simulink model "CessnaCitationCitationIIModel550_Control"  (R2020b)
settings: Solver=FixedStepAuto  StartTime=0.0  StopTime=10.0  FixedStep=1e-12  MinStep=1e-12  RelTol=1
PreLoadFcn:
  | CessnaCitationData
  | datcom_data = datcomimport('Citation.out'); %Datcom data structures
InitFcn:
  | CessnaCitationData
values from neighbouring files (symbols this model uses):
  gnd_alt = -1500    [CessnaCitationData.m]
  inertia = [19990.488, -0.000, 7138.962 ... (first row only)    [CessnaCitationData.m]
  initpos_e = [0 0 -1500]    [CessnaCitationData.m]
  initrotrates_e = [0 0 0]    [CessnaCitationData.m]
  initrpy_e = [0 0 0]    [CessnaCitationData.m]
  initvel_b = [85 0 0]    [CessnaCitationData.m]
  mass = 3175    [CessnaCitationData.m]
  wind_angle_rates = [0 0 0]    [CessnaCitationData.m]
undefined symbols (not defined in the file or in its folder): Earth, m, s, WGS84
libraries: aerolibasang x4, aerolibtransform2 x4, simulink_extras x3, aerolibconvert2 x2, aerolibwind2 x1, aerolibatmos2 x1, shared3dof x1, sharedtransform x1, aerolibadyn x1
settings Model: SimulationMode=accelerator  Creator=pasquale  LastModifiedBy=pasquale
settings SolverCC: AutoInsertRateTranBlk=on

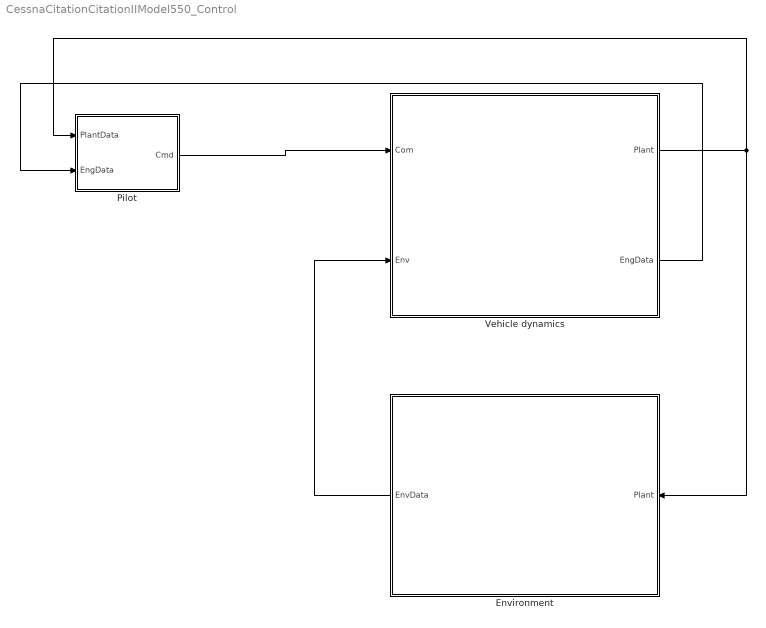
== system CessnaCitationCitationIIModel550_Control ==
  Environment : Subsystem
      mask Display: image('521928855-56a132c45f9b58b7d0bcf732-1.jpg'); % Use "Edit Image" on toolstrip to change.
  Pilot : Subsystem
  Vehicle dynamics : Subsystem
      mask Display: image('Cessna-Citation-II-IISP-S.jpg'); % Use "Edit Image" on toolstrip to change.
  wires:
  Vehicle dynamics/1(Plant) -> Environment/1(Plant), Pilot/1(PlantData)
  Environment/1(EnvData) -> Vehicle dynamics/2(Env)
  Pilot/1(Cmd) -> Vehicle dynamics/1(Com)
  Vehicle dynamics/2(EngData) -> Pilot/2(EngData)

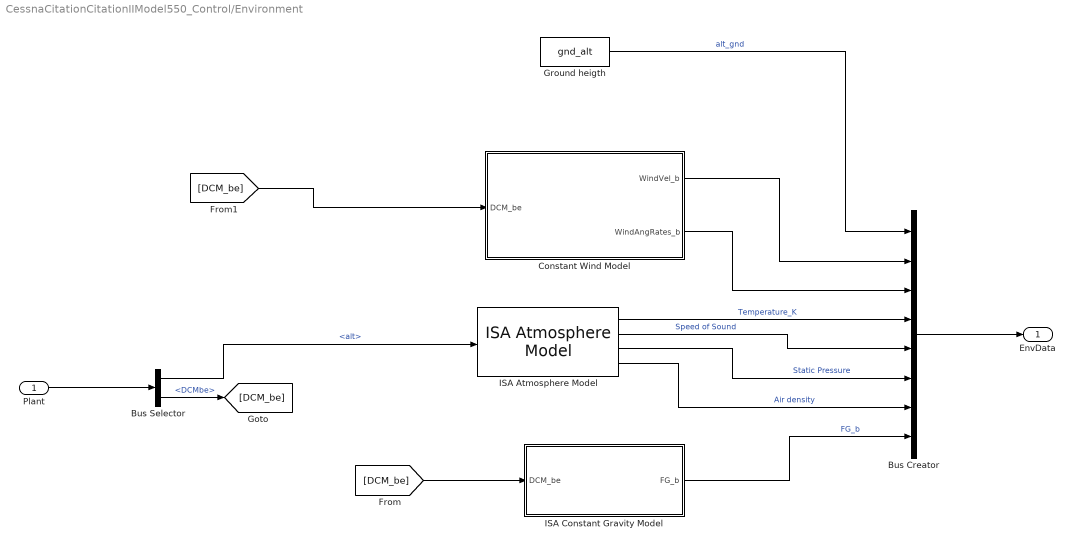
== system CessnaCitationCitationIIModel550_Control/Environment ==
  Plant : Inport
  Bus Creator : BusCreator  Inputs=8
  Bus Selector : BusSelector  OutputSignals=alt,DCMbe
  Constant Wind Model : Subsystem
  Ground heigth : Constant  Value=gnd_alt
  ISA Atmosphere Model : aerolibatmos2/ISA Atmosphere Model  custom=off  g=9.80665  gamma=1.4  R=287.0531  L=0.0065  h_trop=11000  h_strat=20000  rho0=1.225  P0=101325  T0=288.15  h0=0
  ISA Constant Gravity Model : Subsystem
  EnvData : Outport
  wires:
  Plant/1 -> Bus Selector/1
  Bus Selector/1 -> ISA Atmosphere Model/1  "<alt>"
  Bus Creator/1 -> EnvData/1
  ISA Atmosphere Model/4 -> Bus Creator/7  "Air density"
  ISA Atmosphere Model/3 -> Bus Creator/6  "Static Pressure"
  ISA Atmosphere Model/2 -> Bus Creator/5  "Speed of Sound"
  ISA Atmosphere Model/1 -> Bus Creator/4  "Temperature_K"
  Bus Selector/2 -> [DCM_be]  "<DCMbe>"
  [DCM_be] -> Constant Wind Model/1(DCM_be)
  Constant Wind Model/1(WindVel_b) -> Bus Creator/2
  Constant Wind Model/2(WindAngRates_b) -> Bus Creator/3
  ISA Constant Gravity Model/1(FG_b) -> Bus Creator/8  "FG_b"
  [DCM_be] -> ISA Constant Gravity Model/1(DCM_be)
  Ground heigth/1 -> Bus Creator/1  "alt_gnd"

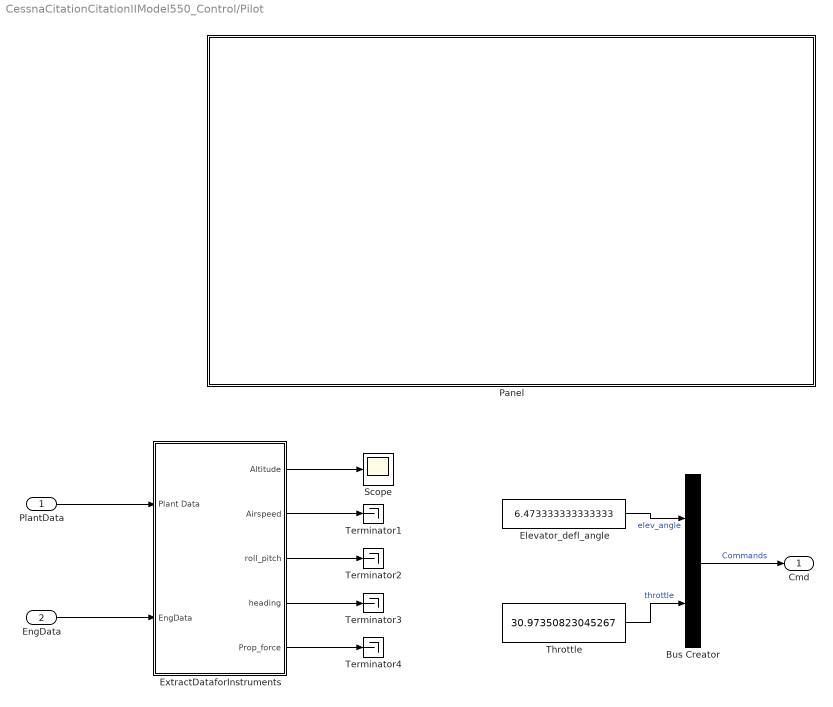
== system CessnaCitationCitationIIModel550_Control/Pilot ==
  PlantData : Inport
  EngData : Inport  Port=2
  Bus Creator : BusCreator  Inputs=2
  Elevator_defl_angle : Constant  Value=6.473333333333333
  ExtractDataforInstruments : Subsystem
  Panel : Subsystem
  Scope : Scope
  Terminator{1..4} (4 alike) : Terminator
  Throttle : Constant  Value=30.97350823045267
  Cmd : Outport
  wires:
  Bus Creator/1 -> Cmd/1  "Commands"
  Elevator_defl_angle/1 -> Bus Creator/1  "elev_angle"
  Throttle/1 -> Bus Creator/2  "throttle"
  PlantData/1 -> ExtractDataforInstruments/1(Plant Data)
  ExtractDataforInstruments/1(Altitude) -> Scope/1
  ExtractDataforInstruments/2(Airspeed) -> Terminator1/1
  ExtractDataforInstruments/3(roll_pitch) -> Terminator2/1
  ExtractDataforInstruments/4(heading) -> Terminator3/1
  ExtractDataforInstruments/5(Prop_force) -> Terminator4/1
  EngData/1 -> ExtractDataforInstruments/2(EngData)

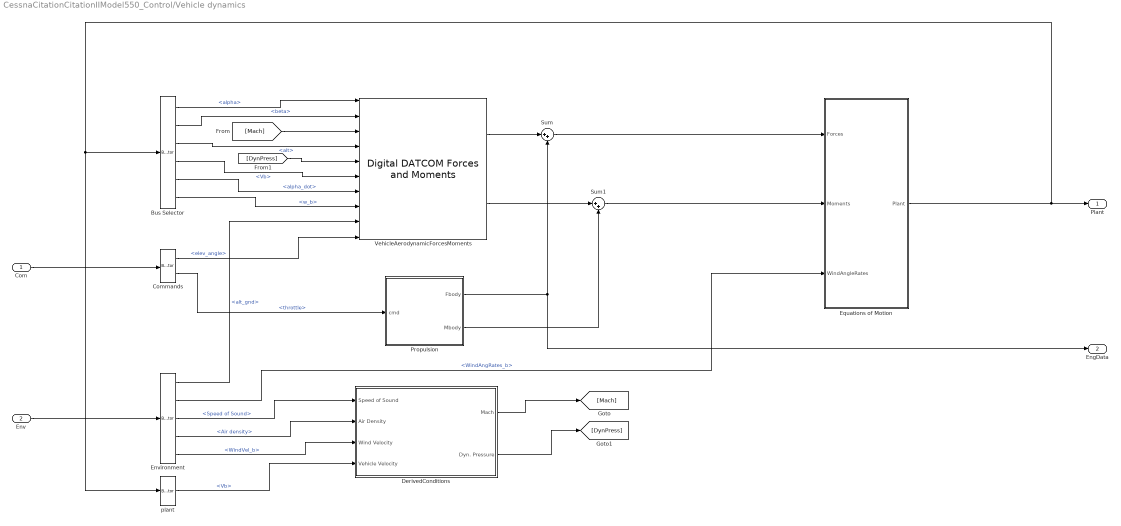
== system CessnaCitationCitationIIModel550_Control/Vehicle dynamics ==
  Com : Inport
  Env : Inport  Port=2
  Bus Selector : BusSelector  OutputSignals=alpha,beta,alt,Vb,alpha_dot,w_b
  Commands : BusSelector  OutputSignals=elev_angle,throttle
  DerivedConditions : Subsystem
  Environment : BusSelector  OutputSignals=alt_gnd,WindAngRates_b,Speed of Sound,Air density,WindVel_b
  Equations of Motion : Subsystem
  Propulsion : Subsystem
  Sum : Sum  Inputs=|++
  Sum1 : Sum  Inputs=|++
  VehicleAerodynamicForcesMoments : aerolibadyn/Digital DATCOM Forces and Moments  units=Metric (MKS)  dcase=datcom_data{3}  fmode=Body  buildno=0  imethod=Linear  emethod=Linear  rmethod=Linear Extrapolation  action=None
      settings: SourceProductBaseCode=AE
  plant : BusSelector  OutputSignals=Vb
  Plant : Outport
  EngData : Outport  Port=2
  wires:
  Propulsion/1(Fbody) -> Sum/2, EngData/1
  Propulsion/2(Mbody) -> Sum1/2
  DerivedConditions/2(Dyn. Pressure) -> [DynPress]
  VehicleAerodynamicForcesMoments/1 -> Sum/1
  DerivedConditions/1(Mach) -> [Mach]
  VehicleAerodynamicForcesMoments/2 -> Sum1/1
  [Mach] -> VehicleAerodynamicForcesMoments/3
  [DynPress] -> VehicleAerodynamicForcesMoments/5
  Bus Selector/2 -> VehicleAerodynamicForcesMoments/2  "<beta>"
  Bus Selector/3 -> VehicleAerodynamicForcesMoments/4  "<alt>"
  Bus Selector/4 -> VehicleAerodynamicForcesMoments/6  "<Vb>"
  Bus Selector/6 -> VehicleAerodynamicForcesMoments/8  "<w_b>"
  plant/1 -> DerivedConditions/4(Vehicle Velocity)  "<Vb>"
  Equations of Motion/1(Plant) -> plant/1, Bus Selector/1, Plant/1
  Sum/1 -> Equations of Motion/1(Forces)
  Sum1/1 -> Equations of Motion/2(Moments)
  Env/1 -> Environment/1
  Com/1 -> Commands/1
  Environment/5 -> DerivedConditions/3(Wind Velocity)  "<WindVel_b>"
  Environment/4 -> DerivedConditions/2(Air Density)  "<Air density>"
  Environment/3 -> DerivedConditions/1(Speed of Sound)  "<Speed of Sound>"
  Environment/2 -> Equations of Motion/3(WindAngleRates)  "<WindAngRates_b>"
  Environment/1 -> VehicleAerodynamicForcesMoments/9  "<alt_gnd>"
  Commands/1 -> VehicleAerodynamicForcesMoments/10  "<elev_angle>"
  Commands/2 -> Propulsion/1(cmd)  "<throttle>"
  Bus Selector/1 -> VehicleAerodynamicForcesMoments/1  "<alpha>"
  Bus Selector/5 -> VehicleAerodynamicForcesMoments/7  "<alpha_dot>"

== system CessnaCitationCitationIIModel550_Control/Environment/Constant Wind Model ==
  DCM_be : Inport
  Horizontal Wind Model : aerolibwind2/Horizontal Wind Model  units=Metric (MKS)  Vw_source=Internal  Vwind=wind_speed  W_source=Internal  Wdeg=wind_dir
      settings: SourceProductBaseCode=AE
  Product2 : Product  Multiplication=Matrix(*)
  Wind_ang_rates : Constant  Value=wind_angle_rates
  WindVel_b : Outport
  WindAngRates_b : Outport  Port=2
  wires:
  DCM_be/1 -> Horizontal Wind Model/1, Product2/1
  Horizontal Wind Model/1 -> WindVel_b/1  "WindVel_b"
  Wind_ang_rates/1 -> Product2/2
  Product2/1 -> WindAngRates_b/1  "WindAngRates_b"

== system CessnaCitationCitationIIModel550_Control/Environment/ISA Constant Gravity Model ==
  DCM_be : Inport
  Gain : Gain  Gain=[0 0 mass]
  ISA constant gravity : Constant  Value=9.80665
  Product : Product  Multiplication=Matrix(*)
  FG_b : Outport
  wires:
  ISA constant gravity/1 -> Gain/1
  Gain/1 -> Product/2  "Fg in flat earth axis"
  DCM_be/1 -> Product/1
  Product/1 -> FG_b/1  "FG_b"

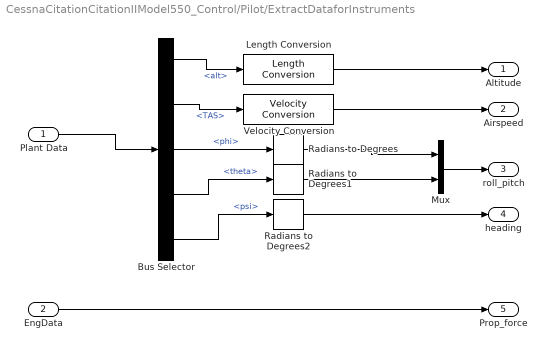
== system CessnaCitationCitationIIModel550_Control/Pilot/ExtractDataforInstruments ==
  Plant Data : Inport
  EngData : Inport  Port=2
  Bus Selector : BusSelector  OutputSignals=alt,TAS,body angles.phi,body angles.theta,body angles.psi
  Length Conversion : aerolibconvert2/Length Conversion  IU=m  OU=ft
  Mux : Mux  Inputs=2
  Radians to Degrees : simulink_extras/Transformations/Radians to Degrees
  Radians to Degrees1 : simulink_extras/Transformations/Radians to Degrees
  Radians to Degrees2 : simulink_extras/Transformations/Radians to Degrees
  Velocity Conversion : aerolibconvert2/Velocity Conversion  IU=m/s  OU=kts
  Altitude : Outport
  Airspeed : Outport  Port=2
  roll_pitch : Outport  Port=3
  heading : Outport  Port=4
  Prop_force : Outport  Port=5
  wires:
  Plant Data/1 -> Bus Selector/1
  Mux/1 -> roll_pitch/1
  Bus Selector/1 -> Length Conversion/1  "<alt>"
  Length Conversion/1 -> Altitude/1
  Bus Selector/2 -> Velocity Conversion/1  "<TAS>"
  Velocity Conversion/1 -> Airspeed/1
  Bus Selector/3 -> Radians to Degrees/1  "<phi>"
  Bus Selector/4 -> Radians to Degrees1/1  "<theta>"
  Radians to Degrees1/1 -> Mux/2
  Radians to Degrees/1 -> Mux/1
  Bus Selector/5 -> Radians to Degrees2/1  "<psi>"
  Radians to Degrees2/1 -> heading/1
  EngData/1 -> Prop_force/1

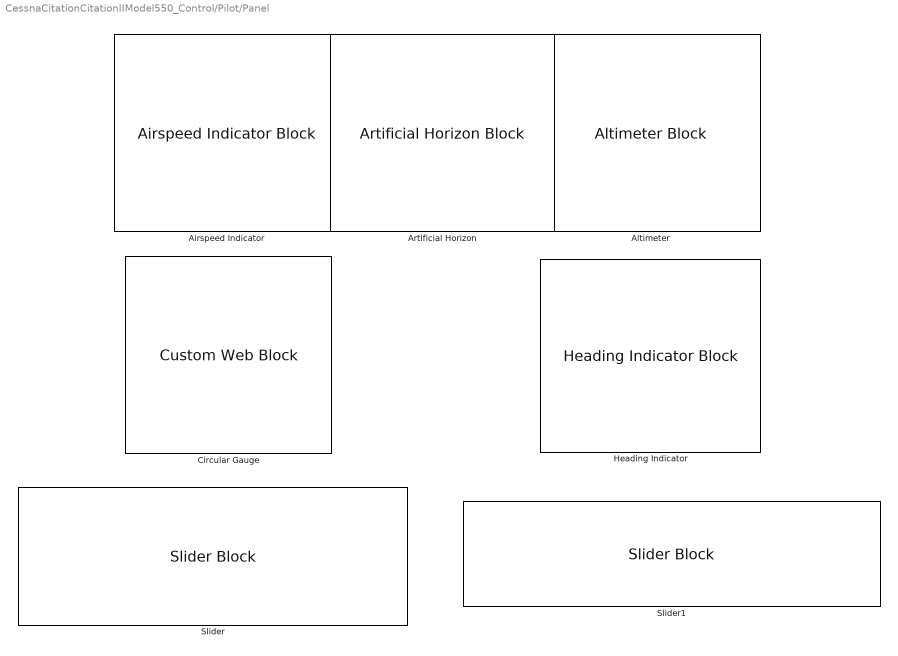
== system CessnaCitationCitationIIModel550_Control/Pilot/Panel ==
  Airspeed Indicator : AirspeedIndicatorBlock  LabelPosition=Hide
  Altimeter : AltimeterBlock  LabelPosition=Hide
  Artificial Horizon : ArtificialHorizonBlock  LabelPosition=Hide
  Circular Gauge : CustomWebBlock  LabelPosition=Hide  ShowInitialText=on  Configuration="{\"components\":[{\"name\":\"CircularScaleComponent\",\"settings\":{\"bounds\":{\"max\":11113.2,\"min\":0,\"tickInterval\":\"auto\"},\"direction\":\"cw\",\"flipLimits\":0,\"innerRadius\":0.75,\"internalTickHeightScaleFactor\":1,\"labelColor\":[255,252,199],\"labelFont\":{\"font\":\"Arial\",\"fontSize\":12},\"labelTransparency\":1,\"minorTickHeightScaleFactor\":0.2,\"needleImage\":{\"size\":[1890,567],\"src\":\"data:image\\/svg+xml;base64,PD94bWwgdmVyc2lvbj0iMS4wIiBlbmNvZGluZz0iVVRGLTgiIHN0YW5kYWxvbmU9Im5vIj8+CjxzdmcKICAgeG1sbnM6ZGM9Imh0dHA6Ly9wdXJsLm9yZy9kYy9lbGVtZW50cy8xLjEvIgogICB4bWxuczpjYz0iaHR0cDovL2NyZWF0aXZlY29tbW9ucy5vcmcvbnMjIgogICB4bWxuczpyZGY9Imh0dHA6Ly93d3cudzMub3JnLzE5OTkvMDIvMjItcmRmLXN5bnRheC1ucyMiCiAgIHhtbG5zOnN2Zz0iaHR0cDovL3d3dy53My5vcmcvMjAwMC9zdmciCiAgIHhtbG5zPSJodHRwOi8vd3d3LnczLm9yZy8yMDAwL3N2ZyIKICAgeG1sbnM6 ...(+4096 chars)\"},\"needleOffset\":[0.1610917094974375,0],\"needleOrientation\":-45,\"needleRotation\":180.59702388394928,\"needleSize\":{\"height\":0.13032601008944536,\"width\":0.416859542883425},\"outerRadius\":0.9,\"position\":[0.06486742424242424,0.05627705627705628,0.8917748917748918,0.8787878787878788],\"scaleAngle\":270,\"scaleAngleOffset\":135,\"scaleColors\":[],\"scaleColorsSize\":0.2,\"scalePosition\":[0,0,1,1],\"showLabels\":1,\"showMinorTicks\":1,\"showSpanLine\":1,\"showTicks\":1,\"tickColor\":[255,255,200],\"tickTransparency\":1,\"valueBarColor\":[0,114,189],\"valueBarPosition\":[0,0,1,1],\"valueBarSize\":0.2,\"valueBarTransparency\":1}},{\"name\":\"BackgroundImageComponent\",\"settings\":{\"image\":{\"size\":[500,500],\"src\":\"data:image\\/svg+xml;base64,PD94bWwgdmVyc2lvbj0iMS4wIiBlbmNvZGluZz0iVVRGLTgiIHN0YW5kYWxvbmU9Im5vIj8+CjxzdmcKICAgeG1sbnM6ZGM9Imh0dHA6Ly9wdXJsLm9yZy9kYy9lbGVtZW50cy8xLjEvIgogICB4bWxuczpjYz0iaHR0cDovL2NyZWF0aXZlY29tbW9ucy5vcmcvbnMjIgogICB4bWxuczpyZGY9Imh0dHA6Ly93d3cudzMub3JnLzE5OTkvMDIvMjItcmRmLXN5bnRheC1ucyMiCiAgIHhtbG5zOnN2Zz0iaHR0cDovL3d3dy53My5vcmcvMjAwMC9zdmciCiAgIHhtbG5zPSJodHRwOi8vd3d3LnczLm9yZy8yMDAwL3N2ZyIKICAgeG1sbnM6 ...(+9964 chars)\"},\"position\":[0,0,1,1],\"scaleMode\":\"0\"}},{\"name\":\"ForegroundImageComponent\",\"settings\":{\"image\":{\"size\":[0,0],\"src\":\"default\",\"srcOrientation\":[]},\"isForeground\":1,\"position\":[0,0,1,1],\"scaleMode\":\"0\"}}],\"settings\":{\"BindingType\":\"signal\",\"aspectRatio\":1.0465116279069768,\"direction\":\"cw\",\"fixedAspectRatio\":\"on\",\"flipLimits\":0,\"orientation\":\"horizontal\"},\"type\":\"CircularGauge\"}"
  Heading Indicator : HeadingIndicatorBlock  LabelPosition=Hide
  Slider : SliderBlock  ScaleMin=-16  ScaleMax=16
  Slider1 : SliderBlock

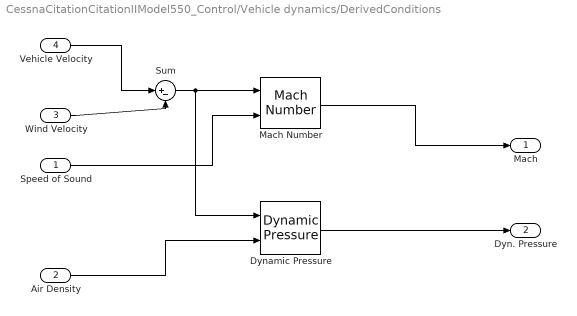
== system CessnaCitationCitationIIModel550_Control/Vehicle dynamics/DerivedConditions ==
  Speed of Sound : Inport
  Air Density : Inport  Port=2
  Wind Velocity : Inport  Port=3
  Vehicle Velocity : Inport  Port=4
  Dynamic Pressure : aerolibasang/Dynamic Pressure
  Mach Number : aerolibasang/Mach Number
      settings: SourceProductBaseCode=AE
  Sum : Sum  Inputs=|+-
  Mach : Outport
  Dyn. Pressure : Outport  Port=2
  wires:
  Vehicle Velocity/1 -> Sum/1
  Wind Velocity/1 -> Sum/2
  Sum/1 -> Dynamic Pressure/1, Mach Number/1
  Speed of Sound/1 -> Mach Number/2
  Mach Number/1 -> Mach/1
  Dynamic Pressure/1 -> Dyn. Pressure/1
  Air Density/1 -> Dynamic Pressure/2

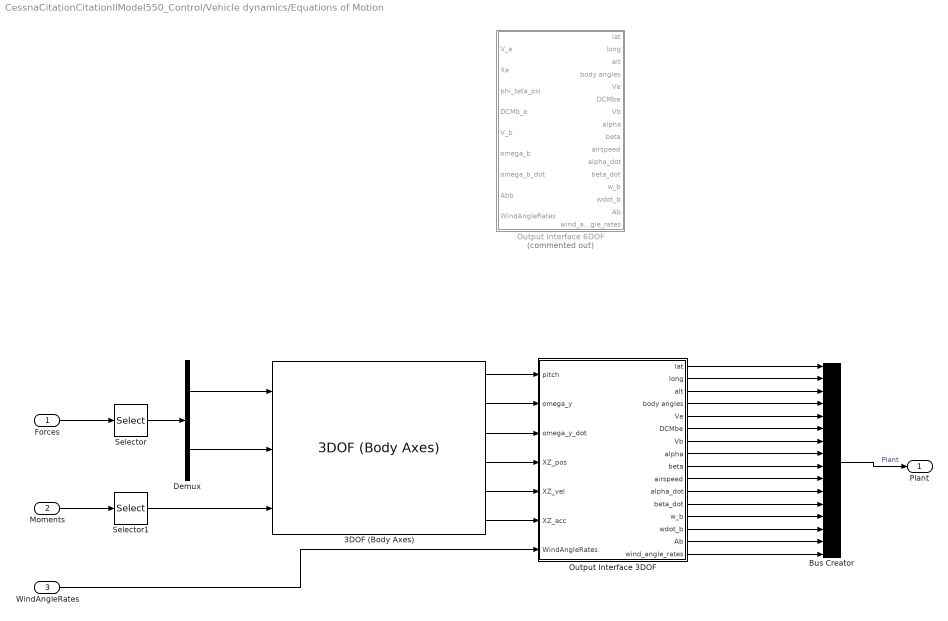
== system CessnaCitationCitationIIModel550_Control/Vehicle dynamics/Equations of Motion ==
  Forces : Inport
  Moments : Inport  Port=2
  WindAngleRates : Inport  Port=3
  3DOF (Body Axes) : shared3dof/3DOF (Body Axes)  units=Metric (MKS)  mtype=Fixed  v_ini=initvel_b(1)  theta_ini=initrpy_e(2)  alpha_ini=0  pos_ini=[initpos_e(1) initpos_e(3)]  q_ini=initrotrates_e(2)  mass=mass  mass_e=0.5  mass_f=3.0  Iyy=inertia(2,2)  Iyy_e=0.5  Iyy_f=3.0  g_in=Internal  g=0  vre_flag=on  abi_flag=off  aMode=0  vel_statename=''  theta_statename=''  pos_statename=''  q_statename=''  mass_statename=''
      settings: SourceProductBaseCode=AE,PW,MT,UV,VE,VP
  Bus Creator : BusCreator  Inputs=16
  Demux : Demux  Outputs=2
  Output Interface 3DOF : Subsystem
  Output Interface 6DOF : Subsystem  Commented=on
  Selector : Selector  InputPortWidth=3  IndexOptions=Index vector (dialog)  Indices=[1 3]  OutputSizes=1
  Selector1 : Selector  InputPortWidth=3  IndexOptions=Index vector (dialog)  Indices=[2]  OutputSizes=1
  Plant : Outport
  wires:
  Bus Creator/1 -> Plant/1  "Plant"
  Forces/1 -> Selector/1
  Demux/1 -> 3DOF (Body Axes)/1
  Demux/2 -> 3DOF (Body Axes)/2
  Selector/1 -> Demux/1
  Moments/1 -> Selector1/1
  Selector1/1 -> 3DOF (Body Axes)/3
  3DOF (Body Axes)/3 -> Output Interface 3DOF/3(omega_y_dot)
  3DOF (Body Axes)/1 -> Output Interface 3DOF/1(pitch)
  3DOF (Body Axes)/2 -> Output Interface 3DOF/2(omega_y)
  3DOF (Body Axes)/4 -> Output Interface 3DOF/4(XZ_pos)
  3DOF (Body Axes)/5 -> Output Interface 3DOF/5(XZ_vel)
  3DOF (Body Axes)/6 -> Output Interface 3DOF/6(XZ_acc)
  Output Interface 3DOF/1(lat) -> Bus Creator/1
  Output Interface 3DOF/2(long) -> Bus Creator/2
  Output Interface 3DOF/3(alt) -> Bus Creator/3
  Output Interface 3DOF/4(body angles) -> Bus Creator/4
  Output Interface 3DOF/5(Ve) -> Bus Creator/5
  Output Interface 3DOF/6(DCMbe) -> Bus Creator/6
  Output Interface 3DOF/7(Vb) -> Bus Creator/7
  Output Interface 3DOF/8(alpha) -> Bus Creator/8
  Output Interface 3DOF/9(beta) -> Bus Creator/9
  Output Interface 3DOF/10(airspeed) -> Bus Creator/10
  Output Interface 3DOF/11(alpha_dot) -> Bus Creator/11
  Output Interface 3DOF/12(beta_dot) -> Bus Creator/12
  Output Interface 3DOF/13(w_b) -> Bus Creator/13
  Output Interface 3DOF/14(wdot_b) -> Bus Creator/14
  Output Interface 3DOF/15(Ab) -> Bus Creator/15
  Output Interface 3DOF/16(wind_angle_rates) -> Bus Creator/16
  WindAngleRates/1 -> Output Interface 3DOF/7(WindAngleRates)

== system CessnaCitationCitationIIModel550_Control/Vehicle dynamics/Propulsion ==
  note: engine is supposed to be on the reference plane of the aircraft, for now
  cmd : Inport
  Ground : Ground
  kg-N conversion : Gain  Gain=9.8
  max thrust [kg] : Gain  Gain=1134
  percent to gain : Gain  Gain=1/100
  Fbody : Outport
  Mbody : Outport  Port=2
  wires:
  percent to gain/1 -> max thrust [kg]/1
  cmd/1 -> percent to gain/1
  max thrust [kg]/1 -> kg-N conversion/1
  kg-N conversion/1 -> Fbody/1
  Ground/1 -> Mbody/1

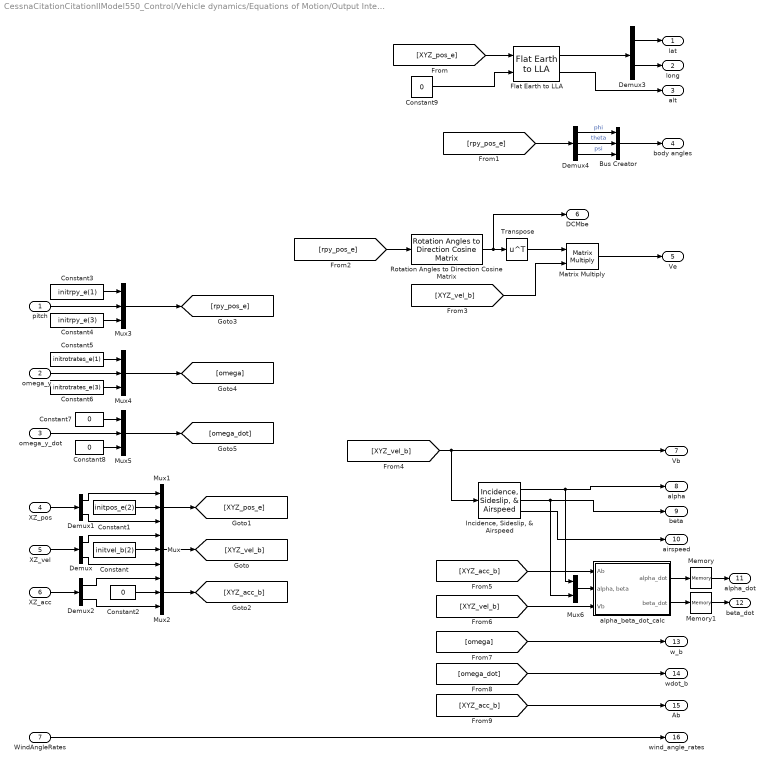
== system CessnaCitationCitationIIModel550_Control/Vehicle dynamics/Equations of Motion/Output Interface 3DOF ==
  pitch : Inport
  omega_y : Inport  Port=2
  omega_y_dot : Inport  Port=3
  XZ_pos : Inport  Port=4
  XZ_vel : Inport  Port=5
  XZ_acc : Inport  Port=6
  WindAngleRates : Inport  Port=7
  Bus Creator : BusCreator  Inputs=3
  Constant : Constant  Value=initvel_b(2)
  Constant1 : Constant  Value=initpos_e(2)
  Constant{2,7..9} (4 alike) : Constant  Value=0
  Constant3 : Constant  Value=initrpy_e(1)
  Constant4 : Constant  Value=initrpy_e(3)
  Constant5 : Constant  Value=initrotrates_e(1)
  Constant6 : Constant  Value=initrotrates_e(3)
  Demux{,1..3} (4 alike) : Demux  Outputs=2
  Demux4 : Demux  Outputs=3
  Flat Earth to LLA : aerolibtransform2/Flat Earth to LLA  units=Metric (MKS)  ptype=Earth (WGS84)  F=1/298.257223563  R=6378137  refPosPort=off  LL0=[0 10]  psi=0
  "Incidence, Sideslip, & Airspeed" : aerolibasang/Incidence, Sideslip, & Airspeed
  Matrix Multiply : Product  Multiplication=Matrix(*)
  Memory : Memory
  Memory1 : Memory
  Mux{,1..5} (6 alike) : Mux  Inputs=3
  Mux6 : Mux  Inputs=2
  Rotation Angles to Direction Cosine Matrix : sharedtransform/Rotation Angles to Direction Cosine Matrix  rotationOrder=ZYX  aMode=aMode
      settings: SourceProductBaseCode=AE,PW,MT,UV,VE,VP
  Transpose : Math  Operator=transpose  SaturateOnIntegerOverflow=on
  alpha_beta_dot_calc : Subsystem
  lat : Outport
  long : Outport  Port=2
  alt : Outport  Port=3
  body angles : Outport  Port=4
  Ve : Outport  Port=5
  DCMbe : Outport  Port=6
  Vb : Outport  Port=7
  alpha : Outport  Port=8
  beta : Outport  Port=9
  airspeed : Outport  Port=10
  alpha_dot : Outport  Port=11
  beta_dot : Outport  Port=12
  w_b : Outport  Port=13
  wdot_b : Outport  Port=14
  Ab : Outport  Port=15
  wind_angle_rates : Outport  Port=16
  wires:
  WindAngleRates/1 -> wind_angle_rates/1
  XZ_vel/1 -> Demux/1
  Constant/1 -> Mux/2
  Demux/1 -> Mux/1
  Demux/2 -> Mux/3
  Mux/1 -> [XYZ_vel_b]
  Mux1/1 -> [XYZ_pos_e]
  Demux1/2 -> Mux1/3
  Demux1/1 -> Mux1/1
  Constant1/1 -> Mux1/2
  XZ_pos/1 -> Demux1/1
  Constant2/1 -> Mux2/2
  Demux2/2 -> Mux2/3
  XZ_acc/1 -> Demux2/1
  Mux2/1 -> [XYZ_acc_b]
  Demux2/1 -> Mux2/1
  pitch/1 -> Mux3/2
  Constant3/1 -> Mux3/1
  Constant4/1 -> Mux3/3
  Mux3/1 -> [rpy_pos_e]
  Mux4/1 -> [omega]
  Constant6/1 -> Mux4/3
  Constant5/1 -> Mux4/1
  omega_y/1 -> Mux4/2
  omega_y_dot/1 -> Mux5/2
  Constant7/1 -> Mux5/1
  Constant8/1 -> Mux5/3
  Mux5/1 -> [omega_dot]
  Demux3/1 -> lat/1
  Demux3/2 -> long/1
  Flat Earth to LLA/1 -> Demux3/1
  Flat Earth to LLA/2 -> alt/1
  [XYZ_pos_e] -> Flat Earth to LLA/1
  Constant9/1 -> Flat Earth to LLA/2
  Demux4/2 -> Bus Creator/2  "theta"
  Demux4/1 -> Bus Creator/1  "phi"
  Demux4/3 -> Bus Creator/3  "psi"
  Bus Creator/1 -> body angles/1
  [rpy_pos_e] -> Demux4/1
  [rpy_pos_e] -> Rotation Angles to Direction Cosine Matrix/1
  Rotation Angles to Direction Cosine Matrix/1 -> DCMbe/1, Transpose/1
  Transpose/1 -> Matrix Multiply/1
  [XYZ_vel_b] -> Matrix Multiply/2
  Matrix Multiply/1 -> Ve/1
  [XYZ_vel_b] -> "Incidence, Sideslip, & Airspeed"/1, Vb/1
  "Incidence, Sideslip, & Airspeed"/1 -> Mux6/1, alpha/1
  "Incidence, Sideslip, & Airspeed"/2 -> Mux6/2, beta/1
  "Incidence, Sideslip, & Airspeed"/3 -> airspeed/1
  alpha_beta_dot_calc/1(alpha_dot) -> Memory/1
  Memory/1 -> alpha_dot/1
  alpha_beta_dot_calc/2(beta_dot) -> Memory1/1
  Memory1/1 -> beta_dot/1
  Mux6/1 -> alpha_beta_dot_calc/2("alpha, beta")
  [XYZ_acc_b] -> alpha_beta_dot_calc/1(Ab)
  [XYZ_vel_b] -> alpha_beta_dot_calc/3(Vb)
  [omega] -> w_b/1
  [omega_dot] -> wdot_b/1
  [XYZ_acc_b] -> Ab/1

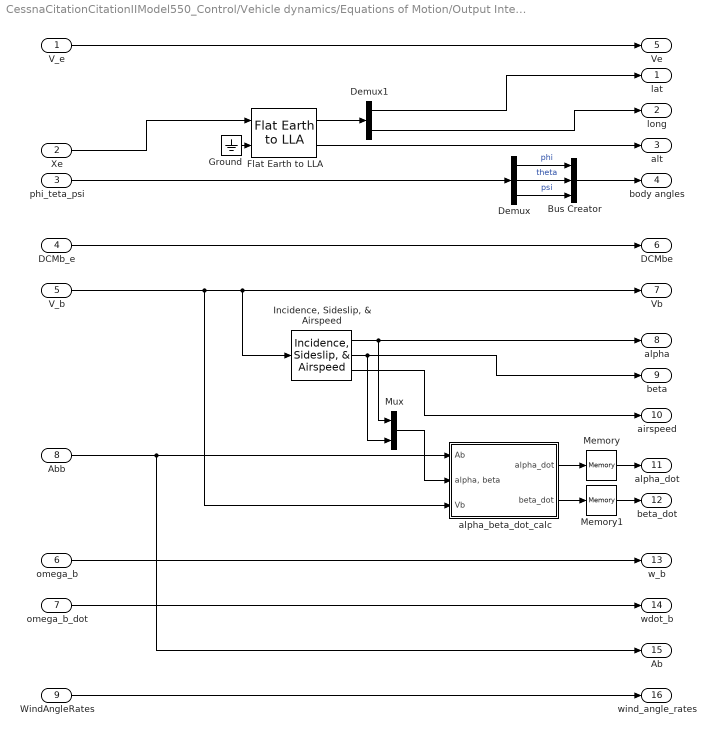
== system CessnaCitationCitationIIModel550_Control/Vehicle dynamics/Equations of Motion/Output Interface 6DOF ==
  V_e : Inport
  Xe : Inport  Port=2
  phi_teta_psi : Inport  Port=3
  DCMb_e : Inport  Port=4
  V_b : Inport  Port=5
  omega_b : Inport  Port=6
  omega_b_dot : Inport  Port=7
  Abb : Inport  Port=8
  WindAngleRates : Inport  Port=9
  Bus Creator : BusCreator  Inputs=3
  Demux : Demux  Outputs=3
  Demux1 : Demux  Outputs=2
  Flat Earth to LLA : aerolibtransform2/Flat Earth to LLA  units=Metric (MKS)  ptype=Earth (WGS84)  F=1/298.257223563  R=6378137  refPosPort=off  LL0=[0 10]  psi=0
  Ground : Ground
  "Incidence, Sideslip, & Airspeed" : aerolibasang/Incidence, Sideslip, & Airspeed
  Memory : Memory
  Memory1 : Memory
  Mux : Mux  Inputs=2
  alpha_beta_dot_calc : Subsystem
  lat : Outport
  long : Outport  Port=2
  alt : Outport  Port=3
  body angles : Outport  Port=4
  Ve : Outport  Port=5
  DCMbe : Outport  Port=6
  Vb : Outport  Port=7
  alpha : Outport  Port=8
  beta : Outport  Port=9
  airspeed : Outport  Port=10
  alpha_dot : Outport  Port=11
  beta_dot : Outport  Port=12
  w_b : Outport  Port=13
  wdot_b : Outport  Port=14
  Ab : Outport  Port=15
  wind_angle_rates : Outport  Port=16
  wires:
  Demux/2 -> Bus Creator/2  "theta"
  Ground/1 -> Flat Earth to LLA/2
  Demux/3 -> Bus Creator/3  "psi"
  Demux1/1 -> lat/1
  Flat Earth to LLA/2 -> alt/1
  Flat Earth to LLA/1 -> Demux1/1
  Demux1/2 -> long/1
  Demux/1 -> Bus Creator/1  "phi"
  Bus Creator/1 -> body angles/1
  phi_teta_psi/1 -> Demux/1
  Xe/1 -> Flat Earth to LLA/1
  DCMb_e/1 -> DCMbe/1
  V_b/1 -> alpha_beta_dot_calc/3(Vb), "Incidence, Sideslip, & Airspeed"/1, Vb/1
  "Incidence, Sideslip, & Airspeed"/1 -> Mux/1, alpha/1
  "Incidence, Sideslip, & Airspeed"/2 -> Mux/2, beta/1
  "Incidence, Sideslip, & Airspeed"/3 -> airspeed/1
  Abb/1 -> Ab/1, alpha_beta_dot_calc/1(Ab)
  Mux/1 -> alpha_beta_dot_calc/2("alpha, beta")
  V_e/1 -> Ve/1
  omega_b/1 -> w_b/1
  omega_b_dot/1 -> wdot_b/1
  WindAngleRates/1 -> wind_angle_rates/1
  alpha_beta_dot_calc/1(alpha_dot) -> Memory/1
  alpha_beta_dot_calc/2(beta_dot) -> Memory1/1
  Memory/1 -> alpha_dot/1
  Memory1/1 -> beta_dot/1

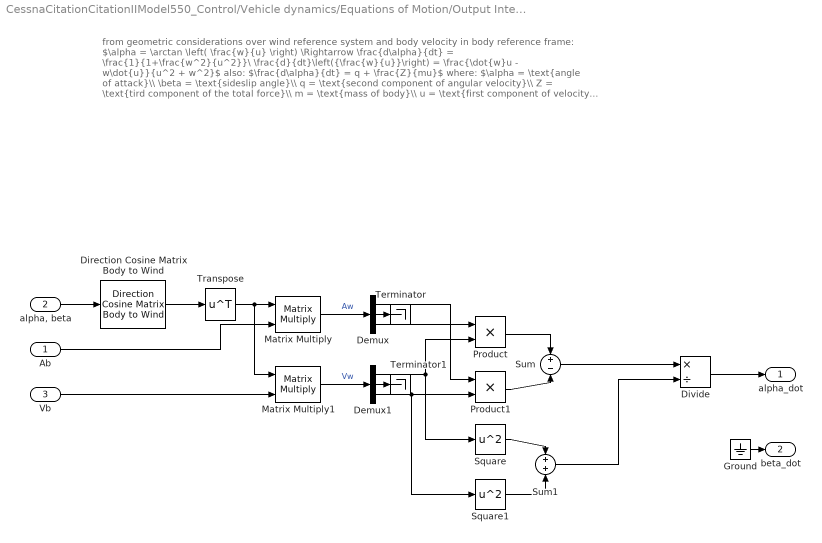
== system CessnaCitationCitationIIModel550_Control/Vehicle dynamics/Equations of Motion/Output Interface 3DOF/alpha_beta_dot_calc ==
  note: from geometric considerations over wind reference system and body velocity in body reference frame:
      | $\alpha = \arctan \left( \frac{w}{u} \right) \Rightarrow \frac{d\alpha}{dt} = \frac{1}{1+\frac{w^2}{u^2}}\ \frac{d}{dt}\left({\frac{w}{u}}\right) = \frac{\dot{w}u - w\dot{u}}{u^2 + w^2}$
      | also:
      | $\frac{d\alpha}{dt} = q + \frac{Z}{mu}$
      | where:
      | $\alpha = \text{angle of attack}\\ \beta = \text{sideslip angle}\\ q = \text{second component of angular velocity}\\ Z = \text{tird component of the total force}\\ m = \text{mass of body}\\ u = \text{first component of velocity in wind reference frame}\\ w = \text{third component of velocity in wind reference frame}$
      |
      | same can be done for $\dot{\beta}$
  Ab : Inport
  "alpha, beta" : Inport  Port=2
  Vb : Inport  Port=3
  Demux : Demux  Outputs=3
  Demux1 : Demux  Outputs=3
  Direction Cosine Matrix Body to Wind : aerolibtransform2/Direction Cosine Matrix Body to Wind
      settings: SourceProductBaseCode=AE
  Divide : Product  Inputs=*/
  Ground : Ground
  Matrix Multiply : Product  Multiplication=Matrix(*)
  Matrix Multiply1 : Product  Multiplication=Matrix(*)
  Product : Product
  Product1 : Product
  Square : Math  Operator=square  SaturateOnIntegerOverflow=on
  Square1 : Math  Operator=square  SaturateOnIntegerOverflow=on
  Sum : Sum  Inputs=+|-
  Sum1 : Sum  Inputs=+|+
  Terminator : Terminator
  Terminator1 : Terminator
  Transpose : Math  Operator=transpose  SaturateOnIntegerOverflow=on
  alpha_dot : Outport
  beta_dot : Outport  Port=2
  wires:
  "alpha, beta"/1 -> Direction Cosine Matrix Body to Wind/1
  Direction Cosine Matrix Body to Wind/1 -> Transpose/1
  Transpose/1 -> Matrix Multiply1/1, Matrix Multiply/1
  Ab/1 -> Matrix Multiply/2
  Vb/1 -> Matrix Multiply1/2
  Matrix Multiply1/1 -> Demux1/1  "Vw"
  Matrix Multiply/1 -> Demux/1  "Aw"
  Demux/3 -> Product/1
  Demux1/1 -> Square/1, Product/2
  Demux1/3 -> Square1/1, Product1/2
  Demux/1 -> Product1/1
  Product/1 -> Sum/1
  Product1/1 -> Sum/2
  Sum/1 -> Divide/1
  Square/1 -> Sum1/1
  Square1/1 -> Sum1/2
  Sum1/1 -> Divide/2
  Divide/1 -> alpha_dot/1
  Ground/1 -> beta_dot/1
  Demux/2 -> Terminator/1
  Demux1/2 -> Terminator1/1

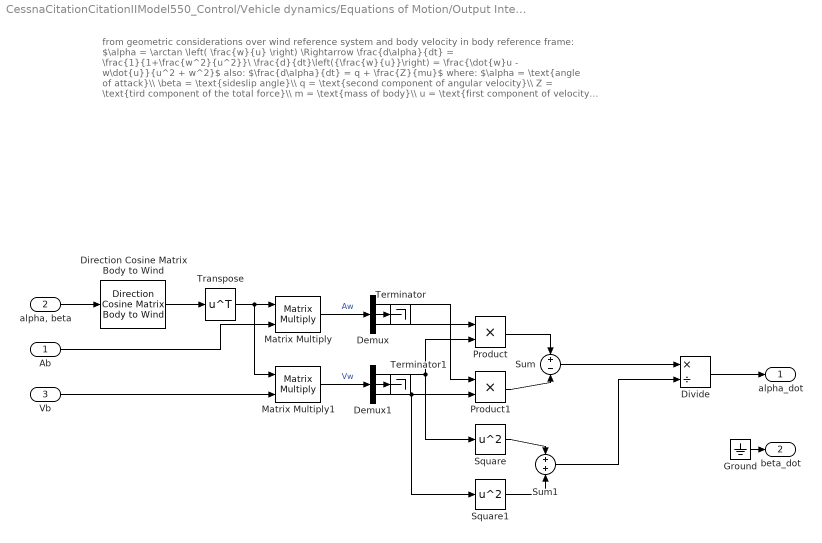
== system CessnaCitationCitationIIModel550_Control/Vehicle dynamics/Equations of Motion/Output Interface 6DOF/alpha_beta_dot_calc ==
  note: from geometric considerations over wind reference system and body velocity in body reference frame:
      | $\alpha = \arctan \left( \frac{w}{u} \right) \Rightarrow \frac{d\alpha}{dt} = \frac{1}{1+\frac{w^2}{u^2}}\ \frac{d}{dt}\left({\frac{w}{u}}\right) = \frac{\dot{w}u - w\dot{u}}{u^2 + w^2}$
      | also:
      | $\frac{d\alpha}{dt} = q + \frac{Z}{mu}$
      | where:
      | $\alpha = \text{angle of attack}\\ \beta = \text{sideslip angle}\\ q = \text{second component of angular velocity}\\ Z = \text{tird component of the total force}\\ m = \text{mass of body}\\ u = \text{first component of velocity in wind reference frame}\\ w = \text{third component of velocity in wind reference frame}$
      |
      | same can be done for $\dot{\beta}$
  Ab : Inport
  "alpha, beta" : Inport  Port=2
  Vb : Inport  Port=3
  Demux : Demux  Outputs=3
  Demux1 : Demux  Outputs=3
  Direction Cosine Matrix Body to Wind : aerolibtransform2/Direction Cosine Matrix Body to Wind
      settings: SourceProductBaseCode=AE
  Divide : Product  Inputs=*/
  Ground : Ground
  Matrix Multiply : Product  Multiplication=Matrix(*)
  Matrix Multiply1 : Product  Multiplication=Matrix(*)
  Product : Product
  Product1 : Product
  Square : Math  Operator=square  SaturateOnIntegerOverflow=on
  Square1 : Math  Operator=square  SaturateOnIntegerOverflow=on
  Sum : Sum  Inputs=+|-
  Sum1 : Sum  Inputs=+|+
  Terminator : Terminator
  Terminator1 : Terminator
  Transpose : Math  Operator=transpose  SaturateOnIntegerOverflow=on
  alpha_dot : Outport
  beta_dot : Outport  Port=2
  wires:
  "alpha, beta"/1 -> Direction Cosine Matrix Body to Wind/1
  Direction Cosine Matrix Body to Wind/1 -> Transpose/1
  Transpose/1 -> Matrix Multiply1/1, Matrix Multiply/1
  Ab/1 -> Matrix Multiply/2
  Vb/1 -> Matrix Multiply1/2
  Matrix Multiply1/1 -> Demux1/1  "Vw"
  Matrix Multiply/1 -> Demux/1  "Aw"
  Demux/3 -> Product/1
  Demux1/1 -> Square/1, Product/2
  Demux1/3 -> Square1/1, Product1/2
  Demux/1 -> Product1/1
  Product/1 -> Sum/1
  Product1/1 -> Sum/2
  Sum/1 -> Divide/1
  Square/1 -> Sum1/1
  Square1/1 -> Sum1/2
  Sum1/1 -> Divide/2
  Divide/1 -> alpha_dot/1
  Ground/1 -> beta_dot/1
  Demux/2 -> Terminator/1
  Demux1/2 -> Terminator1/1
